simulink model "s0405_fmincon"  (R2019b)
settings: Solver=ode1  StartTime=0.0  StopTime=T_sim  FixedStep=dt  RelTol=1e-3
values from neighbouring files (symbols this model uses):
  dt = 1e-4    (= 0.0001)    [m0303_init.m]    (also in m0310_init.m = mean(diff(log.time)); m0312_init.m; m0314_init.m = 0.002; m0318_init.m = 0.0002)
  PARAMS =     [s0310_main.mat]
settings Model: Creator=paolo  LastModifiedBy=opc
settings DebuggingCC: SFMachineParentedDataDiag=error  ArithmeticOperatorsInVariantConditions=warning
settings SFSimCC: CustomCodeUndefinedFunction=UseInterfaceOnly
settings CodeAppCC: StateflowObjectComments=on

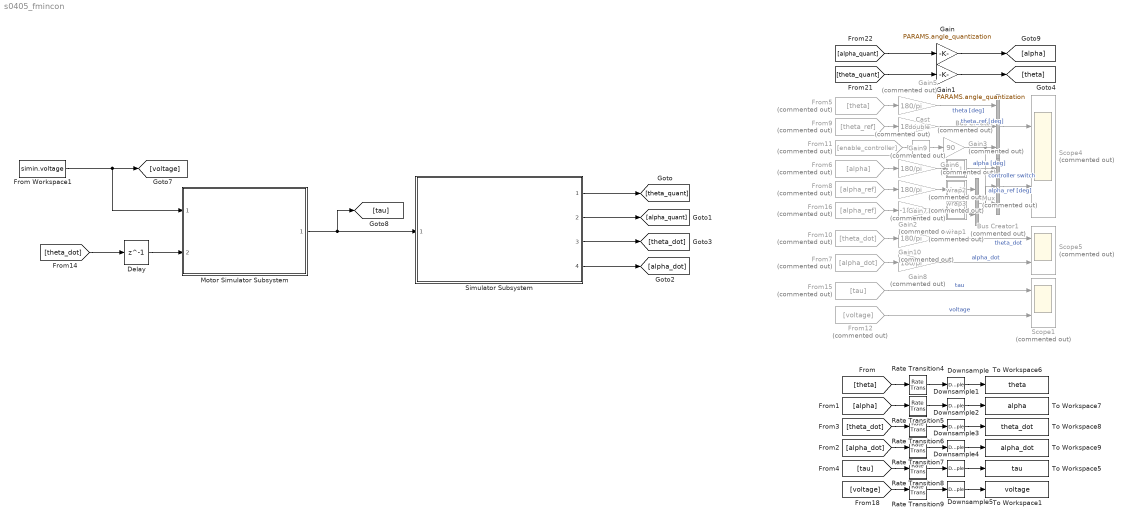
== system s0405_fmincon ==
  Bus Creator : BusCreator  Commented=on  Inputs=3
  Bus Creator1 : BusCreator  Commented=on  Inputs=3
  Cast : DataTypeConversion  Commented=on  OutDataTypeStr=double
  Delay : Delay  DelayLength=1  InitialCondition=PARAMS.th_dot_0
  Downsample{,1..5} (6 alike) : DownSample  N=ceil((2e-3)/dt)  RateOptions=Allow multirate processing
  From Workspace1 : FromWorkspace  VariableName=simin.voltage  SampleTime=0
  From10 : From  Commented=on  GotoTag=theta_dot
  From11 : From  Commented=on  GotoTag=enable_controller
  From12 : From  Commented=on  GotoTag=voltage
  From15 : From  Commented=on  GotoTag=tau
  From16 : From  Commented=on  GotoTag=alpha_ref
  From5 : From  Commented=on  GotoTag=theta
  From6 : From  Commented=on  GotoTag=alpha
  From7 : From  Commented=on  GotoTag=alpha_dot
  From8 : From  Commented=on  GotoTag=alpha_ref
  From9 : From  Commented=on  GotoTag=theta_ref
  Gain : Gain  Gain=PARAMS.angle_quantization
  Gain1 : Gain  Gain=PARAMS.angle_quantization
  Gain{5..10} (6 alike) : Gain  Commented=on  Gain=180/pi
  Gain2 : Gain  Commented=on  Gain=-180/pi
  Gain3 : Gain  Commented=on  Gain=90
  Motor Simulator Subsystem : Subsystem  ReferencedSubsystem=s0303_motor_simulator  omega_0=PARAMS.th_dot_0  i_0=0
  Mux : Mux  Commented=on  Inputs=2
  Rate Transition{4..9} (6 alike) : RateTransition  OutPortSampleTime=dt
  Scope1 : Scope  Commented=on  NumInputPorts=2
  Scope4 : Scope  Commented=on  NumInputPorts=2
  Scope5 : Scope  Commented=on  NumInputPorts=2
  Simulator Subsystem : Subsystem  ReferencedSubsystem=s0405_mechanical_simulator  th_0=PARAMS.th_0  al_0=PARAMS.al_0  th_dot_0=PARAMS.th_dot_0  al_dot_0=PARAMS.al_dot_0
  To Workspace1 : ToWorkspace  VariableName=voltage  SaveFormat=Timeseries  SampleTime=-1
  To Workspace5 : ToWorkspace  VariableName=tau  SaveFormat=Timeseries  SampleTime=-1
  To Workspace6 : ToWorkspace  VariableName=theta  SaveFormat=Timeseries  SampleTime=-1
  To Workspace7 : ToWorkspace  VariableName=alpha  SaveFormat=Timeseries  SampleTime=-1
  To Workspace8 : ToWorkspace  VariableName=theta_dot  SaveFormat=Timeseries  SampleTime=-1
  To Workspace9 : ToWorkspace  VariableName=alpha_dot  SaveFormat=Timeseries  SampleTime=-1
  wrap1 : MATLAB Function  Commented=on  TreatAsAtomicUnit=on
  wrap2 : MATLAB Function  Commented=on  TreatAsAtomicUnit=on
  wrap3 : MATLAB Function  Commented=on  TreatAsAtomicUnit=on
  wires:
  Simulator Subsystem/1 -> [theta_quant]
  Simulator Subsystem/2 -> [alpha_quant]
  Simulator Subsystem/4 -> [alpha_dot]
  Simulator Subsystem/3 -> [theta_dot]
  Motor Simulator Subsystem/1 -> Simulator Subsystem/1, [tau]
  Bus Creator/1 -> Scope4/1
  From8/1 -> Gain7/1
  From5/1 -> Gain5/1
  From6/1 -> Gain6/1
  Gain8/1 -> Scope5/2  "alpha_dot"
  Bus Creator1/1 -> Scope4/2
  From10/1 -> Gain10/1
  From7/1 -> Gain8/1
  Gain10/1 -> Scope5/1  "theta_dot"
  From9/1 -> Gain9/1
  [theta_dot] -> Delay/1
  From12/1 -> Scope1/2  "voltage"
  From15/1 -> Scope1/1  "tau"
  Delay/1 -> Motor Simulator Subsystem/2
  [theta] -> Rate Transition4/1
  [alpha] -> Rate Transition5/1
  [theta_dot] -> Rate Transition6/1
  [alpha_dot] -> Rate Transition7/1
  [tau] -> Rate Transition8/1
  [voltage] -> Rate Transition9/1
  Downsample5/1 -> To Workspace1/1
  Downsample4/1 -> To Workspace5/1
  Downsample3/1 -> To Workspace9/1
  Downsample2/1 -> To Workspace8/1
  Downsample1/1 -> To Workspace7/1
  Downsample/1 -> To Workspace6/1
  Rate Transition4/1 -> Downsample/1
  Rate Transition5/1 -> Downsample1/1
  Rate Transition6/1 -> Downsample2/1
  Rate Transition7/1 -> Downsample3/1
  Rate Transition8/1 -> Downsample4/1
  Rate Transition9/1 -> Downsample5/1
  Gain9/1 -> Bus Creator/2  "theta_ref [deg]"
  wrap2/1(y) -> Bus Creator1/1  "alpha [deg]"
  Gain6/1 -> wrap2/1(u)
  Gain7/1 -> wrap3/1(u)
  Gain5/1 -> Bus Creator/1  "theta [deg]"
  [alpha_quant] -> Gain/1
  Gain/1 -> [alpha]
  Gain1/1 -> [theta]
  [theta_quant] -> Gain1/1
  wrap3/1(y) -> Mux/1
  Mux/1 -> Bus Creator1/2  "alpha_ref [deg]"
  Gain2/1 -> wrap1/1(u)
  From16/1 -> Gain2/1
  wrap1/1(y) -> Mux/2
  From11/1 -> Cast/1
  Gain3/1 -> Bus Creator1/3, Bus Creator/3  "controller switch"
  Cast/1 -> Gain3/1
  From Workspace1/1 -> Motor Simulator Subsystem/1, [voltage]

== matlab function s0405_fmincon/wrap2 ==
  data: u input; y output
function y = wrap(u)
stop_condition = false;
y = u;
while ~stop_condition
    if y > 270
        y = y - 360;
    elseif y < -270
        y = y + 360;
    else
        stop_condition = true;
    end
end

== matlab function s0405_fmincon/wrap3 ==
  data: u input; y output
function y = wrap(u)
stop_condition = false;
y = u;
while ~stop_condition
    if y > 270
        y = y - 360;
    elseif y < -270
        y = y + 360;
    else
        stop_condition = true;
    end
end

== matlab function s0405_fmincon/wrap1 ==
  data: u input; y output
function y = wrap(u)
stop_condition = false;
y = u;
while ~stop_condition
    if y > 270
        y = y - 360;
    elseif y < -270
        y = y + 360;
    else
        stop_condition = true;
    end
end
